simulink model "CSTR_sim_old"  (R2017a)
settings: Solver=ode8  StartTime=0.0  StopTime=t_end  FixedStep=Ts  RelTol=1e-3
values from neighbouring files (symbols this model uses):
  A1 = Kss.A    [decentralized_control.m]    (also in decentralized_simulation.m)
  A2 = Kss.A    [decoupling_dc_simulation.m]
  A3 = Kss.A    [decoupling_w0_simulation.m]
  A4 = Kss.A    [h_inf_simulation.m]
  A5 = Kss.A    [inversion_simulation.m]
  B1 = Kss.B    [decentralized_control.m]    (also in decentralized_simulation.m)
  B2 = Kss.B    [decoupling_dc_simulation.m]
  B3 = Kss.B    [decoupling_w0_simulation.m]
  B4 = Kss.B    [h_inf_simulation.m]
  B5 = Kss.B    [inversion_simulation.m]
  C1 = Kss.C    [decentralized_control.m]    (also in decentralized_simulation.m; dencentralizovano.m = [1 0; 0 1])
  C2 = Kss.C    [decoupling_dc_simulation.m]
  C3 = Kss.C    [decoupling_w0_simulation.m]
  C4 = Kss.C    [h_inf_simulation.m]
  C5 = Kss.C    [inversion_simulation.m]
  Ca = 1e-6    (= 1e-06)    [initialisation.m]    (also in linearisation.m = m.Ca; parameters.mat)
  Cb = 1e-6    (= 1e-06)    [initialisation.m]    (also in linearisation.m = m.Cb; parameters.mat)
  D1 = Kss.D    [decentralized_control.m]    (also in decentralized_simulation.m)
  D2 = Kss.D    [decoupling_dc_simulation.m]
  D3 = Kss.D    [decoupling_w0_simulation.m]
  D4 = Kss.D    [h_inf_simulation.m]
  D5 = Kss.D    [inversion_simulation.m]
  Fa0 = double(eval(S.Fa))    [linearisation.m]    (also in set_point.mat = 0.00260416666667)
  Fb0 = double(eval(S.Fb))    [linearisation.m]    (also in set_point.mat = 0.00572916666667)
  K_sel = 1    [decentralized_simulation.m]    (also in decoupling_dc_simulation.m = 2; decoupling_w0_simulation.m = 3; h_inf_simulation.m = 4; inversion_simulation.m = 5)
  kv = 0.01    [initialisation.m]    (also in linearisation.m = m.kv; parameters.mat)
  kw = 1e-14    [initialisation.m]    (also in linearisation.m = m.kw; parameters.mat)
  V = 30    [initialisation.m]    (also in linearisation.m = m.V; parameters.mat)
  xa0 = 3.1250e-07    (= 3.125e-07)    [initialisation.m]    (also in linearisation.m = m.xa0; parameters.mat; set_point.mat)
  y0 = m.y    [linearisation.m]    (also in set_point.mat = 7)
undefined symbols (not defined in the file or in its folder): d1, d2, tFa_d_down, tFa_d_up, tFb_d_down, tFb_d_up, txa_d_down, txa_r_up, ty_r_down, ty_r_up
settings Model: Creator=Ivona  LastModifiedBy=Milosh Yokich
settings SimscapeCC: SimscapeNormalizeSystem=off

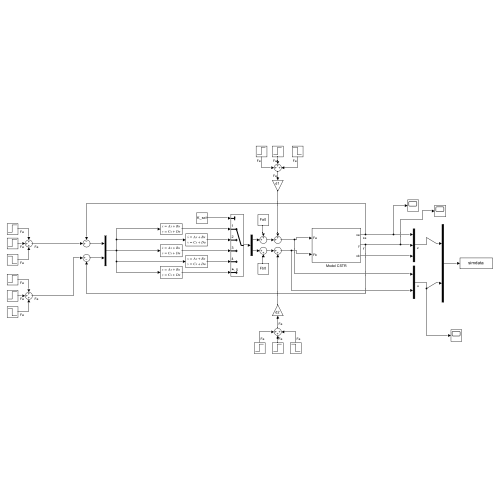
[thumbnail: Simulink's stored preview of the top-level diagram]
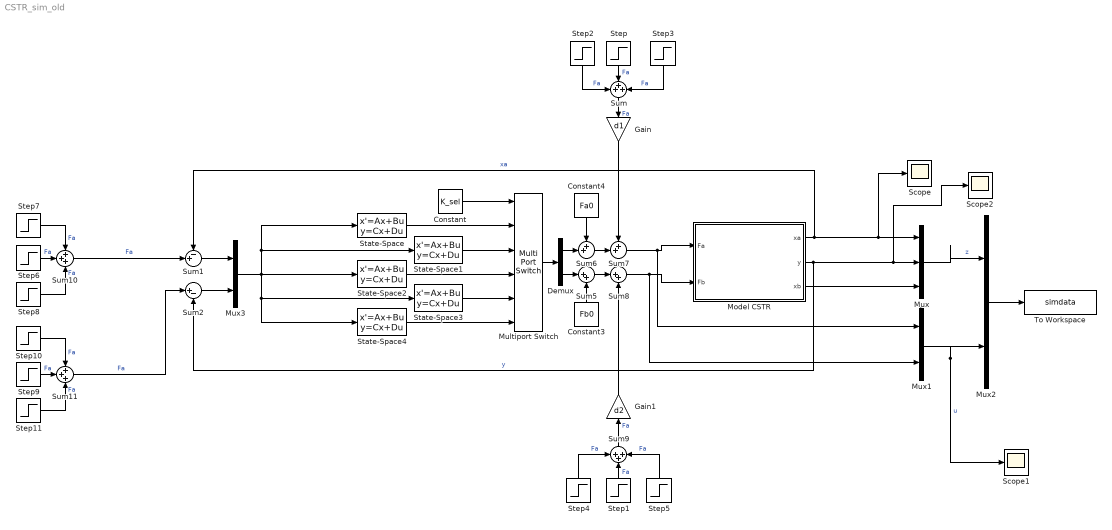
== system CSTR_sim_old ==
  Constant : Constant  Value=K_sel
  Constant3 : Constant  Value=Fb0
  Constant4 : Constant  Value=Fa0
  Demux : Demux  Outputs=2
  Gain : Gain  Gain=d1
  Gain1 : Gain  Gain=d2
  Model CSTR : Subsystem
  Multiport Switch : MultiPortSwitch  Inputs=5
  Mux : Mux  Inputs=3
  Mux1 : Mux  Inputs=2
  Mux2 : Mux  Inputs=2
  Mux3 : Mux  Inputs=2
  Scope : Scope
  Scope1 : Scope
  Scope2 : Scope
  State-Space : StateSpace  A=A1  B=B1  C=C1  D=D1  X0=0
  State-Space1 : StateSpace  A=A2  B=B2  C=C2  D=D2  X0=0
  State-Space2 : StateSpace  A=A3  B=B3  C=C3  D=D3  X0=0
  State-Space3 : StateSpace  A=A4  B=B4  C=C4  D=D4  X0=0
  State-Space4 : StateSpace  A=A5  B=B5  C=C5  D=D5  X0=0
  Step : Step  Time=0  After=0  SampleTime=0
  Step1 : Step  Time=0  After=0  SampleTime=0
  Step10 : Step  Time=ty_r_up  After=0.1*y0  SampleTime=0
  Step11 : Step  Time=ty_r_down  After=-0.1*y0  SampleTime=0
  Step2 : Step  Time=tFa_d_up  After=0.1*Fa0  SampleTime=0
  Step3 : Step  Time=tFa_d_down  After=-0.1*Fa0  SampleTime=0
  Step4 : Step  Time=tFb_d_up  After=0.1*Fb0  SampleTime=0
  Step5 : Step  Time=tFb_d_down  After=-0.1*Fb0  SampleTime=0
  Step6 : Step  Time=0  After=xa0  SampleTime=0
  Step7 : Step  Time=txa_r_up  After=0.1*xa0  SampleTime=0
  Step8 : Step  Time=txa_d_down  After=-0.1*xa0  SampleTime=0
  Step9 : Step  Time=0  After=y0  SampleTime=0
  Sum{,9..11} (4 alike) : Sum  Inputs=+++
  Sum1 : Sum  Inputs=-+|
  Sum2 : Sum  Inputs=|+-
  Sum5 : Sum  Inputs=|++
  Sum6 : Sum  Inputs=++|
  Sum7 : Sum  Inputs=++|
  Sum8 : Sum  Inputs=|++
  To Workspace : ToWorkspace  VariableName=simdata  SaveFormat=Timeseries  SampleTime=-1
  wires:
  Model CSTR/1(xa) -> Sum1/1, Mux/1, Scope/1  "xa"
  Model CSTR/2(y) -> Sum2/2, Mux/2, Scope2/1  "y"
  Mux/1 -> Mux2/1  "z"
  Mux1/1 -> Scope1/1, Mux2/2  "u"
  Mux2/1 -> To Workspace/1
  Step/1 -> Sum/2  "Fa"
  Step2/1 -> Sum/1  "Fa"
  Step3/1 -> Sum/3  "Fa"
  Model CSTR/3(xb) -> Mux/3
  Multiport Switch/1 -> Demux/1
  State-Space/1 -> Multiport Switch/2
  State-Space1/1 -> Multiport Switch/3
  State-Space2/1 -> Multiport Switch/4
  State-Space3/1 -> Multiport Switch/5
  State-Space4/1 -> Multiport Switch/6
  Constant/1 -> Multiport Switch/1
  Mux3/1 -> State-Space4/1, State-Space3/1, State-Space1/1, State-Space/1, State-Space2/1
  Sum1/1 -> Mux3/1
  Sum2/1 -> Mux3/2
  Demux/2 -> Sum5/1
  Demux/1 -> Sum6/2
  Constant3/1 -> Sum5/2
  Constant4/1 -> Sum6/1
  Sum6/1 -> Sum7/2
  Gain/1 -> Sum7/1
  Sum5/1 -> Sum8/1
  Sum7/1 -> Mux1/1, Model CSTR/1(Fa)
  Sum8/1 -> Mux1/2, Model CSTR/2(Fb)
  Gain1/1 -> Sum8/2
  Sum/1 -> Gain/1  "Fa"
  Step4/1 -> Sum9/1  "Fa"
  Step1/1 -> Sum9/2  "Fa"
  Step5/1 -> Sum9/3  "Fa"
  Sum9/1 -> Gain1/1  "Fa"
  Step7/1 -> Sum10/1  "Fa"
  Step6/1 -> Sum10/2  "Fa"
  Step8/1 -> Sum10/3  "Fa"
  Sum10/1 -> Sum1/2  "Fa"
  Step10/1 -> Sum11/1  "Fa"
  Step9/1 -> Sum11/2  "Fa"
  Step11/1 -> Sum11/3  "Fa"
  Sum11/1 -> Sum2/1  "Fa"

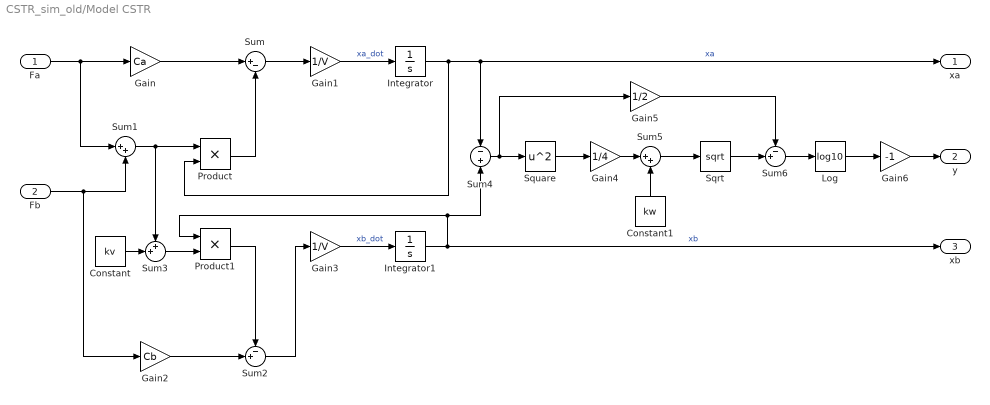
== system CSTR_sim_old/Model CSTR ==
  Fa : Inport
  Fb : Inport  Port=2
  Constant : Constant  Value=kv
  Constant1 : Constant  Value=kw
  Gain : Gain  Gain=Ca
  Gain1 : Gain  Gain=1/V
  Gain2 : Gain  Gain=Cb
  Gain3 : Gain  Gain=1/V
  Gain4 : Gain  Gain=1/4
  Gain5 : Gain  Gain=1/2
  Gain6 : Gain  Gain=-1
  Integrator : Integrator
  Integrator1 : Integrator
  Log : Math  Operator=log10  SaturateOnIntegerOverflow=on
  Product : Product
  Product1 : Product
  Sqrt : Sqrt  SaturateOnIntegerOverflow=on
  Square : Math  Operator=square  SaturateOnIntegerOverflow=on
  Sum : Sum  Inputs=|+-
  Sum1 : Sum  Inputs=|++
  Sum2 : Sum  Inputs=-+|
  Sum3 : Sum  Inputs=++|
  Sum4 : Sum  Inputs=-+
  Sum5 : Sum  Inputs=|++
  Sum6 : Sum  Inputs=-+|
  xa : Outport
  y : Outport  Port=2
  xb : Outport  Port=3
  wires:
  Integrator/1 -> Product/2, Sum4/1, xa/1  "xa"
  Fa/1 -> Sum1/1, Gain/1
  Gain/1 -> Sum/1
  Fb/1 -> Gain2/1, Sum1/2
  Sum1/1 -> Sum3/1, Product/1
  Product/1 -> Sum/2
  Sum/1 -> Gain1/1
  Gain1/1 -> Integrator/1  "xa_dot"
  Gain2/1 -> Sum2/2
  Constant/1 -> Sum3/2
  Product1/1 -> Sum2/1
  Sum2/1 -> Gain3/1
  Integrator1/1 -> xb/1, Sum4/2, Product1/1  "xb"
  Sum3/1 -> Product1/2
  Gain3/1 -> Integrator1/1  "xb_dot"
  Square/1 -> Gain4/1
  Gain4/1 -> Sum5/1
  Constant1/1 -> Sum5/2
  Sum5/1 -> Sqrt/1
  Sqrt/1 -> Sum6/2
  Gain5/1 -> Sum6/1
  Sum6/1 -> Log/1
  Log/1 -> Gain6/1
  Gain6/1 -> y/1
  Sum4/1 -> Gain5/1, Square/1
